simulink model "TrajectoryGenerator3DOF"  (R2023b)
settings: Solver=FixedStepDiscrete  StartTime=0.0  StopTime=1.364*1.4  FixedStep=0.002  RelTol=1e-3
undefined symbols (not defined in the file or in its folder): M_z, Smoothers, Ts
(part 2 of 4)

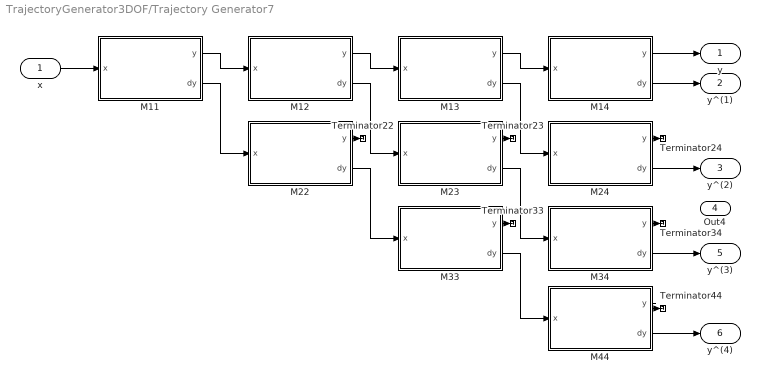
== system TrajectoryGenerator3DOF/Trajectory Generator7 ==
  x : Inport
  M11 : Subsystem  AncestorBlock=Smoothers/M_z  mask{N=643, Ts=0.002, Q0=0}
      mask prompts: N "N_i"; Ts "Sampling period (Ts)"; Q0 "Initial position"
  M12 : Subsystem  AncestorBlock=Smoothers/M_z  mask{N=429, Ts=0.002, Q0=0}
      mask prompts: N "N_i"; Ts "Sampling period (Ts)"; Q0 "Initial position"
  M13 : Subsystem  AncestorBlock=Smoothers/M_z  mask{N=215, Ts=0.002, Q0=0}
      mask prompts: N "N_i"; Ts "Sampling period (Ts)"; Q0 "Initial position"
  M14 : Subsystem  AncestorBlock=Smoothers/M_z  mask{N=215, Ts=0.002, Q0=0}
      mask prompts: N "N_i"; Ts "Sampling period (Ts)"; Q0 "Initial position"
  M22 : Subsystem  AncestorBlock=Smoothers/M_z  mask{N=429, Ts=0.002, Q0=0}
      mask prompts: N "N_i"; Ts "Sampling period (Ts)"; Q0 "Initial position"
  M23 : Subsystem  AncestorBlock=Smoothers/M_z  mask{N=215, Ts=0.002, Q0=0}
      mask prompts: N "N_i"; Ts "Sampling period (Ts)"; Q0 "Initial position"
  M24 : Subsystem  AncestorBlock=Smoothers/M_z  mask{N=215, Ts=0.002, Q0=0}
      mask prompts: N "N_i"; Ts "Sampling period (Ts)"; Q0 "Initial position"
  M33 : Subsystem  AncestorBlock=Smoothers/M_z  mask{N=215, Ts=0.002, Q0=0}
      mask prompts: N "N_i"; Ts "Sampling period (Ts)"; Q0 "Initial position"
  M34 : Subsystem  AncestorBlock=Smoothers/M_z  mask{N=215, Ts=0.002, Q0=0}
      mask prompts: N "N_i"; Ts "Sampling period (Ts)"; Q0 "Initial position"
  M44 : Subsystem  AncestorBlock=Smoothers/M_z  mask{N=215, Ts=0.002, Q0=0}
      mask prompts: N "N_i"; Ts "Sampling period (Ts)"; Q0 "Initial position"
  Terminator{22..24,33..34,44} (6 alike) : Terminator
  y : Outport
  y^(1) : Outport  Port=2
  y^(2) : Outport  Port=3
  Out4 : Outport  Port=4
  y^(3) : Outport  Port=5
  y^(4) : Outport  Port=6
  wires:
  x/1 -> M11/1(x)
  M11/1(y) -> M12/1(x)
  M12/1(y) -> M13/1(x)
  M13/1(y) -> M14/1(x)
  M11/2(dy) -> M22/1(x)
  M12/2(dy) -> M23/1(x)
  M13/2(dy) -> M24/1(x)
  M22/2(dy) -> M33/1(x)
  M23/2(dy) -> M34/1(x)
  M33/2(dy) -> M44/1(x)
  M22/1(y) -> Terminator22/1
  M23/1(y) -> Terminator23/1
  M24/1(y) -> Terminator24/1
  M33/1(y) -> Terminator33/1
  M34/1(y) -> Terminator34/1
  M44/1(y) -> Terminator44/1
  M14/1(y) -> y/1
  M14/2(dy) -> y^(1)/1
  M24/2(dy) -> y^(2)/1
  M34/2(dy) -> y^(3)/1
  M44/2(dy) -> y^(4)/1

== system TrajectoryGenerator3DOF/Trajectory Generator8 ==
  x : Inport
  M11 : Subsystem  AncestorBlock=Smoothers/M_z  mask{N=166, Ts=0.002, Q0=0}
      mask prompts: N "N_i"; Ts "Sampling period (Ts)"; Q0 "Initial position"
  M12 : Subsystem  AncestorBlock=Smoothers/M_z  mask{N=86, Ts=0.002, Q0=0}
      mask prompts: N "N_i"; Ts "Sampling period (Ts)"; Q0 "Initial position"
  M13 : Subsystem  AncestorBlock=Smoothers/M_z  mask{N=43, Ts=0.002, Q0=0}
      mask prompts: N "N_i"; Ts "Sampling period (Ts)"; Q0 "Initial position"
  M14 : Subsystem  AncestorBlock=Smoothers/M_z  mask{N=43, Ts=0.002, Q0=0}
      mask prompts: N "N_i"; Ts "Sampling period (Ts)"; Q0 "Initial position"
  M22 : Subsystem  AncestorBlock=Smoothers/M_z  mask{N=86, Ts=0.002, Q0=0}
      mask prompts: N "N_i"; Ts "Sampling period (Ts)"; Q0 "Initial position"
  M23 : Subsystem  AncestorBlock=Smoothers/M_z  mask{N=43, Ts=0.002, Q0=0}
      mask prompts: N "N_i"; Ts "Sampling period (Ts)"; Q0 "Initial position"
  M24 : Subsystem  AncestorBlock=Smoothers/M_z  mask{N=43, Ts=0.002, Q0=0}
      mask prompts: N "N_i"; Ts "Sampling period (Ts)"; Q0 "Initial position"
  M33 : Subsystem  AncestorBlock=Smoothers/M_z  mask{N=43, Ts=0.002, Q0=0}
      mask prompts: N "N_i"; Ts "Sampling period (Ts)"; Q0 "Initial position"
  M34 : Subsystem  AncestorBlock=Smoothers/M_z  mask{N=43, Ts=0.002, Q0=0}
      mask prompts: N "N_i"; Ts "Sampling period (Ts)"; Q0 "Initial position"
  M44 : Subsystem  AncestorBlock=Smoothers/M_z  mask{N=43, Ts=0.002, Q0=0}
      mask prompts: N "N_i"; Ts "Sampling period (Ts)"; Q0 "Initial position"
  Terminator{22..24,33..34,44} (6 alike) : Terminator
  y : Outport
  y^(1) : Outport  Port=2
  y^(2) : Outport  Port=3
  y^(3) : Outport  Port=4
  y^(4) : Outport  Port=5
  wires:
  x/1 -> M11/1(x)
  M11/1(y) -> M12/1(x)
  M12/1(y) -> M13/1(x)
  M13/1(y) -> M14/1(x)
  M11/2(dy) -> M22/1(x)
  M12/2(dy) -> M23/1(x)
  M13/2(dy) -> M24/1(x)
  M22/2(dy) -> M33/1(x)
  M23/2(dy) -> M34/1(x)
  M33/2(dy) -> M44/1(x)
  M22/1(y) -> Terminator22/1
  M23/1(y) -> Terminator23/1
  M24/1(y) -> Terminator24/1
  M33/1(y) -> Terminator33/1
  M34/1(y) -> Terminator34/1
  M44/1(y) -> Terminator44/1
  M14/1(y) -> y/1
  M14/2(dy) -> y^(1)/1
  M24/2(dy) -> y^(2)/1
  M34/2(dy) -> y^(3)/1
  M44/2(dy) -> y^(4)/1

== system TrajectoryGenerator3DOF/Trajectory Generator9 ==
  x : Inport
  M11 : Subsystem  AncestorBlock=Smoothers/M_z  mask{N=193, Ts=0.002, Q0=0}
      mask prompts: N "N_i"; Ts "Sampling period (Ts)"; Q0 "Initial position"
  M12 : Subsystem  AncestorBlock=Smoothers/M_z  mask{N=166, Ts=0.002, Q0=0}
      mask prompts: N "N_i"; Ts "Sampling period (Ts)"; Q0 "Initial position"
  M13 : Subsystem  AncestorBlock=Smoothers/M_z  mask{N=65, Ts=0.002, Q0=0}
      mask prompts: N "N_i"; Ts "Sampling period (Ts)"; Q0 "Initial position"
  M14 : Subsystem  AncestorBlock=Smoothers/M_z  mask{N=65, Ts=0.002, Q0=0}
      mask prompts: N "N_i"; Ts "Sampling period (Ts)"; Q0 "Initial position"
  M22 : Subsystem  AncestorBlock=Smoothers/M_z  mask{N=166, Ts=0.002, Q0=0}
      mask prompts: N "N_i"; Ts "Sampling period (Ts)"; Q0 "Initial position"
  M23 : Subsystem  AncestorBlock=Smoothers/M_z  mask{N=65, Ts=0.002, Q0=0}
      mask prompts: N "N_i"; Ts "Sampling period (Ts)"; Q0 "Initial position"
  M24 : Subsystem  AncestorBlock=Smoothers/M_z  mask{N=65, Ts=0.002, Q0=0}
      mask prompts: N "N_i"; Ts "Sampling period (Ts)"; Q0 "Initial position"
  M33 : Subsystem  AncestorBlock=Smoothers/M_z  mask{N=65, Ts=0.002, Q0=0}
      mask prompts: N "N_i"; Ts "Sampling period (Ts)"; Q0 "Initial position"
  M34 : Subsystem  AncestorBlock=Smoothers/M_z  mask{N=65, Ts=0.002, Q0=0}
      mask prompts: N "N_i"; Ts "Sampling period (Ts)"; Q0 "Initial position"
  M44 : Subsystem  AncestorBlock=Smoothers/M_z  mask{N=65, Ts=0.002, Q0=0}
      mask prompts: N "N_i"; Ts "Sampling period (Ts)"; Q0 "Initial position"
  Terminator{22..24,33..34,44} (6 alike) : Terminator
  y : Outport
  y^(1) : Outport  Port=2
  y^(2) : Outport  Port=3
  y^(3) : Outport  Port=4
  y^(4) : Outport  Port=5
  wires:
  x/1 -> M11/1(x)
  M11/1(y) -> M12/1(x)
  M12/1(y) -> M13/1(x)
  M13/1(y) -> M14/1(x)
  M11/2(dy) -> M22/1(x)
  M12/2(dy) -> M23/1(x)
  M13/2(dy) -> M24/1(x)
  M22/2(dy) -> M33/1(x)
  M23/2(dy) -> M34/1(x)
  M33/2(dy) -> M44/1(x)
  M22/1(y) -> Terminator22/1
  M23/1(y) -> Terminator23/1
  M24/1(y) -> Terminator24/1
  M33/1(y) -> Terminator33/1
  M34/1(y) -> Terminator34/1
  M44/1(y) -> Terminator44/1
  M14/1(y) -> y/1
  M14/2(dy) -> y^(1)/1
  M24/2(dy) -> y^(2)/1
  M34/2(dy) -> y^(3)/1
  M44/2(dy) -> y^(4)/1

== system TrajectoryGenerator3DOF/Trajectory Generator/M11 ==
  x : Inport
  Discrete FIR Filter1 : DiscreteFir  Coefficients=1/N/Ts*[1 zeros(1,N-1) -1]  InitialStates=Q0  SampleTime=Ts
  Discrete Filter : DiscreteFilter  Numerator=[0 Ts]  Denominator=[1 -1]  InitialStates=Q0  SampleTime=Ts
  y : Outport
  dy : Outport  Port=2
  wires:
  Discrete FIR Filter1/1 -> Discrete Filter/1, dy/1
  x/1 -> Discrete FIR Filter1/1
  Discrete Filter/1 -> y/1

== system TrajectoryGenerator3DOF/Trajectory Generator/M12 ==
  x : Inport
  Discrete FIR Filter1 : DiscreteFir  Coefficients=1/N/Ts*[1 zeros(1,N-1) -1]  InitialStates=Q0  SampleTime=Ts
  Discrete Filter : DiscreteFilter  Numerator=[0 Ts]  Denominator=[1 -1]  InitialStates=Q0  SampleTime=Ts
  y : Outport
  dy : Outport  Port=2
  wires:
  Discrete FIR Filter1/1 -> Discrete Filter/1, dy/1
  x/1 -> Discrete FIR Filter1/1
  Discrete Filter/1 -> y/1

== system TrajectoryGenerator3DOF/Trajectory Generator/M13 ==
  x : Inport
  Discrete FIR Filter1 : DiscreteFir  Coefficients=1/N/Ts*[1 zeros(1,N-1) -1]  InitialStates=Q0  SampleTime=Ts
  Discrete Filter : DiscreteFilter  Numerator=[0 Ts]  Denominator=[1 -1]  InitialStates=Q0  SampleTime=Ts
  y : Outport
  dy : Outport  Port=2
  wires:
  Discrete FIR Filter1/1 -> Discrete Filter/1, dy/1
  x/1 -> Discrete FIR Filter1/1
  Discrete Filter/1 -> y/1

== system TrajectoryGenerator3DOF/Trajectory Generator/M14 ==
  x : Inport
  Discrete FIR Filter1 : DiscreteFir  Coefficients=1/N/Ts*[1 zeros(1,N-1) -1]  InitialStates=Q0  SampleTime=Ts
  Discrete Filter : DiscreteFilter  Numerator=[0 Ts]  Denominator=[1 -1]  InitialStates=Q0  SampleTime=Ts
  y : Outport
  dy : Outport  Port=2
  wires:
  Discrete FIR Filter1/1 -> Discrete Filter/1, dy/1
  x/1 -> Discrete FIR Filter1/1
  Discrete Filter/1 -> y/1

== system TrajectoryGenerator3DOF/Trajectory Generator/M22 ==
  x : Inport
  Discrete FIR Filter1 : DiscreteFir  Coefficients=1/N/Ts*[1 zeros(1,N-1) -1]  InitialStates=Q0  SampleTime=Ts
  Discrete Filter : DiscreteFilter  Numerator=[0 Ts]  Denominator=[1 -1]  InitialStates=Q0  SampleTime=Ts
  y : Outport
  dy : Outport  Port=2
  wires:
  Discrete FIR Filter1/1 -> Discrete Filter/1, dy/1
  x/1 -> Discrete FIR Filter1/1
  Discrete Filter/1 -> y/1

== system TrajectoryGenerator3DOF/Trajectory Generator/M23 ==
  x : Inport
  Discrete FIR Filter1 : DiscreteFir  Coefficients=1/N/Ts*[1 zeros(1,N-1) -1]  InitialStates=Q0  SampleTime=Ts
  Discrete Filter : DiscreteFilter  Numerator=[0 Ts]  Denominator=[1 -1]  InitialStates=Q0  SampleTime=Ts
  y : Outport
  dy : Outport  Port=2
  wires:
  Discrete FIR Filter1/1 -> Discrete Filter/1, dy/1
  x/1 -> Discrete FIR Filter1/1
  Discrete Filter/1 -> y/1

== system TrajectoryGenerator3DOF/Trajectory Generator/M24 ==
  x : Inport
  Discrete FIR Filter1 : DiscreteFir  Coefficients=1/N/Ts*[1 zeros(1,N-1) -1]  InitialStates=Q0  SampleTime=Ts
  Discrete Filter : DiscreteFilter  Numerator=[0 Ts]  Denominator=[1 -1]  InitialStates=Q0  SampleTime=Ts
  y : Outport
  dy : Outport  Port=2
  wires:
  Discrete FIR Filter1/1 -> Discrete Filter/1, dy/1
  x/1 -> Discrete FIR Filter1/1
  Discrete Filter/1 -> y/1

== system TrajectoryGenerator3DOF/Trajectory Generator/M33 ==
  x : Inport
  Discrete FIR Filter1 : DiscreteFir  Coefficients=1/N/Ts*[1 zeros(1,N-1) -1]  InitialStates=Q0  SampleTime=Ts
  Discrete Filter : DiscreteFilter  Numerator=[0 Ts]  Denominator=[1 -1]  InitialStates=Q0  SampleTime=Ts
  y : Outport
  dy : Outport  Port=2
  wires:
  Discrete FIR Filter1/1 -> Discrete Filter/1, dy/1
  x/1 -> Discrete FIR Filter1/1
  Discrete Filter/1 -> y/1

== system TrajectoryGenerator3DOF/Trajectory Generator/M34 ==
  x : Inport
  Discrete FIR Filter1 : DiscreteFir  Coefficients=1/N/Ts*[1 zeros(1,N-1) -1]  InitialStates=Q0  SampleTime=Ts
  Discrete Filter : DiscreteFilter  Numerator=[0 Ts]  Denominator=[1 -1]  InitialStates=Q0  SampleTime=Ts
  y : Outport
  dy : Outport  Port=2
  wires:
  Discrete FIR Filter1/1 -> Discrete Filter/1, dy/1
  x/1 -> Discrete FIR Filter1/1
  Discrete Filter/1 -> y/1

== system TrajectoryGenerator3DOF/Trajectory Generator/M44 ==
  x : Inport
  Discrete FIR Filter1 : DiscreteFir  Coefficients=1/N/Ts*[1 zeros(1,N-1) -1]  InitialStates=Q0  SampleTime=Ts
  Discrete Filter : DiscreteFilter  Numerator=[0 Ts]  Denominator=[1 -1]  InitialStates=Q0  SampleTime=Ts
  y : Outport
  dy : Outport  Port=2
  wires:
  Discrete FIR Filter1/1 -> Discrete Filter/1, dy/1
  x/1 -> Discrete FIR Filter1/1
  Discrete Filter/1 -> y/1

== system TrajectoryGenerator3DOF/Trajectory Generator1/M11 ==
  x : Inport
  Discrete FIR Filter1 : DiscreteFir  Coefficients=1/N/Ts*[1 zeros(1,N-1) -1]  InitialStates=Q0  SampleTime=Ts
  Discrete Filter : DiscreteFilter  Numerator=[0 Ts]  Denominator=[1 -1]  InitialStates=Q0  SampleTime=Ts
  y : Outport
  dy : Outport  Port=2
  wires:
  Discrete Filter/1 -> y/1
  x/1 -> Discrete FIR Filter1/1
  Discrete FIR Filter1/1 -> dy/1, Discrete Filter/1

== system TrajectoryGenerator3DOF/Trajectory Generator1/M12 ==
  x : Inport
  Discrete FIR Filter1 : DiscreteFir  Coefficients=1/N/Ts*[1 zeros(1,N-1) -1]  InitialStates=Q0  SampleTime=Ts
  Discrete Filter : DiscreteFilter  Numerator=[0 Ts]  Denominator=[1 -1]  InitialStates=Q0  SampleTime=Ts
  y : Outport
  dy : Outport  Port=2
  wires:
  Discrete Filter/1 -> y/1
  x/1 -> Discrete FIR Filter1/1
  Discrete FIR Filter1/1 -> dy/1, Discrete Filter/1

== system TrajectoryGenerator3DOF/Trajectory Generator1/M13 ==
  x : Inport
  Discrete FIR Filter1 : DiscreteFir  Coefficients=1/N/Ts*[1 zeros(1,N-1) -1]  InitialStates=Q0  SampleTime=Ts
  Discrete Filter : DiscreteFilter  Numerator=[0 Ts]  Denominator=[1 -1]  InitialStates=Q0  SampleTime=Ts
  y : Outport
  dy : Outport  Port=2
  wires:
  Discrete Filter/1 -> y/1
  x/1 -> Discrete FIR Filter1/1
  Discrete FIR Filter1/1 -> dy/1, Discrete Filter/1

== system TrajectoryGenerator3DOF/Trajectory Generator1/M14 ==
  x : Inport
  Discrete FIR Filter1 : DiscreteFir  Coefficients=1/N/Ts*[1 zeros(1,N-1) -1]  InitialStates=Q0  SampleTime=Ts
  Discrete Filter : DiscreteFilter  Numerator=[0 Ts]  Denominator=[1 -1]  InitialStates=Q0  SampleTime=Ts
  y : Outport
  dy : Outport  Port=2
  wires:
  Discrete Filter/1 -> y/1
  x/1 -> Discrete FIR Filter1/1
  Discrete FIR Filter1/1 -> dy/1, Discrete Filter/1

== system TrajectoryGenerator3DOF/Trajectory Generator1/M22 ==
  x : Inport
  Discrete FIR Filter1 : DiscreteFir  Coefficients=1/N/Ts*[1 zeros(1,N-1) -1]  InitialStates=Q0  SampleTime=Ts
  Discrete Filter : DiscreteFilter  Numerator=[0 Ts]  Denominator=[1 -1]  InitialStates=Q0  SampleTime=Ts
  y : Outport
  dy : Outport  Port=2
  wires:
  Discrete Filter/1 -> y/1
  x/1 -> Discrete FIR Filter1/1
  Discrete FIR Filter1/1 -> dy/1, Discrete Filter/1

== system TrajectoryGenerator3DOF/Trajectory Generator1/M23 ==
  x : Inport
  Discrete FIR Filter1 : DiscreteFir  Coefficients=1/N/Ts*[1 zeros(1,N-1) -1]  InitialStates=Q0  SampleTime=Ts
  Discrete Filter : DiscreteFilter  Numerator=[0 Ts]  Denominator=[1 -1]  InitialStates=Q0  SampleTime=Ts
  y : Outport
  dy : Outport  Port=2
  wires:
  Discrete Filter/1 -> y/1
  x/1 -> Discrete FIR Filter1/1
  Discrete FIR Filter1/1 -> dy/1, Discrete Filter/1

== system TrajectoryGenerator3DOF/Trajectory Generator1/M24 ==
  x : Inport
  Discrete FIR Filter1 : DiscreteFir  Coefficients=1/N/Ts*[1 zeros(1,N-1) -1]  InitialStates=Q0  SampleTime=Ts
  Discrete Filter : DiscreteFilter  Numerator=[0 Ts]  Denominator=[1 -1]  InitialStates=Q0  SampleTime=Ts
  y : Outport
  dy : Outport  Port=2
  wires:
  Discrete Filter/1 -> y/1
  x/1 -> Discrete FIR Filter1/1
  Discrete FIR Filter1/1 -> dy/1, Discrete Filter/1

== system TrajectoryGenerator3DOF/Trajectory Generator1/M33 ==
  x : Inport
  Discrete FIR Filter1 : DiscreteFir  Coefficients=1/N/Ts*[1 zeros(1,N-1) -1]  InitialStates=Q0  SampleTime=Ts
  Discrete Filter : DiscreteFilter  Numerator=[0 Ts]  Denominator=[1 -1]  InitialStates=Q0  SampleTime=Ts
  y : Outport
  dy : Outport  Port=2
  wires:
  Discrete Filter/1 -> y/1
  x/1 -> Discrete FIR Filter1/1
  Discrete FIR Filter1/1 -> dy/1, Discrete Filter/1

== system TrajectoryGenerator3DOF/Trajectory Generator1/M34 ==
  x : Inport
  Discrete FIR Filter1 : DiscreteFir  Coefficients=1/N/Ts*[1 zeros(1,N-1) -1]  InitialStates=Q0  SampleTime=Ts
  Discrete Filter : DiscreteFilter  Numerator=[0 Ts]  Denominator=[1 -1]  InitialStates=Q0  SampleTime=Ts
  y : Outport
  dy : Outport  Port=2
  wires:
  Discrete Filter/1 -> y/1
  x/1 -> Discrete FIR Filter1/1
  Discrete FIR Filter1/1 -> dy/1, Discrete Filter/1

== system TrajectoryGenerator3DOF/Trajectory Generator1/M44 ==
  x : Inport
  Discrete FIR Filter1 : DiscreteFir  Coefficients=1/N/Ts*[1 zeros(1,N-1) -1]  InitialStates=Q0  SampleTime=Ts
  Discrete Filter : DiscreteFilter  Numerator=[0 Ts]  Denominator=[1 -1]  InitialStates=Q0  SampleTime=Ts
  y : Outport
  dy : Outport  Port=2
  wires:
  Discrete Filter/1 -> y/1
  x/1 -> Discrete FIR Filter1/1
  Discrete FIR Filter1/1 -> dy/1, Discrete Filter/1

== system TrajectoryGenerator3DOF/Trajectory Generator10/M11 ==
  x : Inport
  Discrete FIR Filter1 : DiscreteFir  Coefficients=1/N/Ts*[1 zeros(1,N-1) -1]  InitialStates=Q0  SampleTime=Ts
  Discrete Filter : DiscreteFilter  Numerator=[0 Ts]  Denominator=[1 -1]  InitialStates=Q0  SampleTime=Ts
  y : Outport
  dy : Outport  Port=2
  wires:
  Discrete FIR Filter1/1 -> Discrete Filter/1, dy/1
  x/1 -> Discrete FIR Filter1/1
  Discrete Filter/1 -> y/1

== system TrajectoryGenerator3DOF/Trajectory Generator10/M12 ==
  x : Inport
  Discrete FIR Filter1 : DiscreteFir  Coefficients=1/N/Ts*[1 zeros(1,N-1) -1]  InitialStates=Q0  SampleTime=Ts
  Discrete Filter : DiscreteFilter  Numerator=[0 Ts]  Denominator=[1 -1]  InitialStates=Q0  SampleTime=Ts
  y : Outport
  dy : Outport  Port=2
  wires:
  Discrete FIR Filter1/1 -> Discrete Filter/1, dy/1
  x/1 -> Discrete FIR Filter1/1
  Discrete Filter/1 -> y/1

== system TrajectoryGenerator3DOF/Trajectory Generator10/M13 ==
  x : Inport
  Discrete FIR Filter1 : DiscreteFir  Coefficients=1/N/Ts*[1 zeros(1,N-1) -1]  InitialStates=Q0  SampleTime=Ts
  Discrete Filter : DiscreteFilter  Numerator=[0 Ts]  Denominator=[1 -1]  InitialStates=Q0  SampleTime=Ts
  y : Outport
  dy : Outport  Port=2
  wires:
  Discrete FIR Filter1/1 -> Discrete Filter/1, dy/1
  x/1 -> Discrete FIR Filter1/1
  Discrete Filter/1 -> y/1

== system TrajectoryGenerator3DOF/Trajectory Generator10/M14 ==
  x : Inport
  Discrete FIR Filter1 : DiscreteFir  Coefficients=1/N/Ts*[1 zeros(1,N-1) -1]  InitialStates=Q0  SampleTime=Ts
  Discrete Filter : DiscreteFilter  Numerator=[0 Ts]  Denominator=[1 -1]  InitialStates=Q0  SampleTime=Ts
  y : Outport
  dy : Outport  Port=2
  wires:
  Discrete FIR Filter1/1 -> Discrete Filter/1, dy/1
  x/1 -> Discrete FIR Filter1/1
  Discrete Filter/1 -> y/1

== system TrajectoryGenerator3DOF/Trajectory Generator10/M22 ==
  x : Inport
  Discrete FIR Filter1 : DiscreteFir  Coefficients=1/N/Ts*[1 zeros(1,N-1) -1]  InitialStates=Q0  SampleTime=Ts
  Discrete Filter : DiscreteFilter  Numerator=[0 Ts]  Denominator=[1 -1]  InitialStates=Q0  SampleTime=Ts
  y : Outport
  dy : Outport  Port=2
  wires:
  Discrete FIR Filter1/1 -> Discrete Filter/1, dy/1
  x/1 -> Discrete FIR Filter1/1
  Discrete Filter/1 -> y/1

== system TrajectoryGenerator3DOF/Trajectory Generator10/M23 ==
  x : Inport
  Discrete FIR Filter1 : DiscreteFir  Coefficients=1/N/Ts*[1 zeros(1,N-1) -1]  InitialStates=Q0  SampleTime=Ts
  Discrete Filter : DiscreteFilter  Numerator=[0 Ts]  Denominator=[1 -1]  InitialStates=Q0  SampleTime=Ts
  y : Outport
  dy : Outport  Port=2
  wires:
  Discrete FIR Filter1/1 -> Discrete Filter/1, dy/1
  x/1 -> Discrete FIR Filter1/1
  Discrete Filter/1 -> y/1

== system TrajectoryGenerator3DOF/Trajectory Generator10/M24 ==
  x : Inport
  Discrete FIR Filter1 : DiscreteFir  Coefficients=1/N/Ts*[1 zeros(1,N-1) -1]  InitialStates=Q0  SampleTime=Ts
  Discrete Filter : DiscreteFilter  Numerator=[0 Ts]  Denominator=[1 -1]  InitialStates=Q0  SampleTime=Ts
  y : Outport
  dy : Outport  Port=2
  wires:
  Discrete FIR Filter1/1 -> Discrete Filter/1, dy/1
  x/1 -> Discrete FIR Filter1/1
  Discrete Filter/1 -> y/1

== system TrajectoryGenerator3DOF/Trajectory Generator10/M33 ==
  x : Inport
  Discrete FIR Filter1 : DiscreteFir  Coefficients=1/N/Ts*[1 zeros(1,N-1) -1]  InitialStates=Q0  SampleTime=Ts
  Discrete Filter : DiscreteFilter  Numerator=[0 Ts]  Denominator=[1 -1]  InitialStates=Q0  SampleTime=Ts
  y : Outport
  dy : Outport  Port=2
  wires:
  Discrete FIR Filter1/1 -> Discrete Filter/1, dy/1
  x/1 -> Discrete FIR Filter1/1
  Discrete Filter/1 -> y/1

== system TrajectoryGenerator3DOF/Trajectory Generator10/M34 ==
  x : Inport
  Discrete FIR Filter1 : DiscreteFir  Coefficients=1/N/Ts*[1 zeros(1,N-1) -1]  InitialStates=Q0  SampleTime=Ts
  Discrete Filter : DiscreteFilter  Numerator=[0 Ts]  Denominator=[1 -1]  InitialStates=Q0  SampleTime=Ts
  y : Outport
  dy : Outport  Port=2
  wires:
  Discrete FIR Filter1/1 -> Discrete Filter/1, dy/1
  x/1 -> Discrete FIR Filter1/1
  Discrete Filter/1 -> y/1

== system TrajectoryGenerator3DOF/Trajectory Generator10/M44 ==
  x : Inport
  Discrete FIR Filter1 : DiscreteFir  Coefficients=1/N/Ts*[1 zeros(1,N-1) -1]  InitialStates=Q0  SampleTime=Ts
  Discrete Filter : DiscreteFilter  Numerator=[0 Ts]  Denominator=[1 -1]  InitialStates=Q0  SampleTime=Ts
  y : Outport
  dy : Outport  Port=2
  wires:
  Discrete FIR Filter1/1 -> Discrete Filter/1, dy/1
  x/1 -> Discrete FIR Filter1/1
  Discrete Filter/1 -> y/1

== system TrajectoryGenerator3DOF/Trajectory Generator11/M11 ==
  x : Inport
  Discrete FIR Filter1 : DiscreteFir  Coefficients=1/N/Ts*[1 zeros(1,N-1) -1]  InitialStates=Q0  SampleTime=Ts
  Discrete Filter : DiscreteFilter  Numerator=[0 Ts]  Denominator=[1 -1]  InitialStates=Q0  SampleTime=Ts
  y : Outport
  dy : Outport  Port=2
  wires:
  Discrete FIR Filter1/1 -> Discrete Filter/1, dy/1
  x/1 -> Discrete FIR Filter1/1
  Discrete Filter/1 -> y/1

== system TrajectoryGenerator3DOF/Trajectory Generator11/M12 ==
  x : Inport
  Discrete FIR Filter1 : DiscreteFir  Coefficients=1/N/Ts*[1 zeros(1,N-1) -1]  InitialStates=Q0  SampleTime=Ts
  Discrete Filter : DiscreteFilter  Numerator=[0 Ts]  Denominator=[1 -1]  InitialStates=Q0  SampleTime=Ts
  y : Outport
  dy : Outport  Port=2
  wires:
  Discrete FIR Filter1/1 -> Discrete Filter/1, dy/1
  x/1 -> Discrete FIR Filter1/1
  Discrete Filter/1 -> y/1

== system TrajectoryGenerator3DOF/Trajectory Generator11/M13 ==
  x : Inport
  Discrete FIR Filter1 : DiscreteFir  Coefficients=1/N/Ts*[1 zeros(1,N-1) -1]  InitialStates=Q0  SampleTime=Ts
  Discrete Filter : DiscreteFilter  Numerator=[0 Ts]  Denominator=[1 -1]  InitialStates=Q0  SampleTime=Ts
  y : Outport
  dy : Outport  Port=2
  wires:
  Discrete FIR Filter1/1 -> Discrete Filter/1, dy/1
  x/1 -> Discrete FIR Filter1/1
  Discrete Filter/1 -> y/1

== system TrajectoryGenerator3DOF/Trajectory Generator11/M14 ==
  x : Inport
  Discrete FIR Filter1 : DiscreteFir  Coefficients=1/N/Ts*[1 zeros(1,N-1) -1]  InitialStates=Q0  SampleTime=Ts
  Discrete Filter : DiscreteFilter  Numerator=[0 Ts]  Denominator=[1 -1]  InitialStates=Q0  SampleTime=Ts
  y : Outport
  dy : Outport  Port=2
  wires:
  Discrete FIR Filter1/1 -> Discrete Filter/1, dy/1
  x/1 -> Discrete FIR Filter1/1
  Discrete Filter/1 -> y/1

== system TrajectoryGenerator3DOF/Trajectory Generator11/M22 ==
  x : Inport
  Discrete FIR Filter1 : DiscreteFir  Coefficients=1/N/Ts*[1 zeros(1,N-1) -1]  InitialStates=Q0  SampleTime=Ts
  Discrete Filter : DiscreteFilter  Numerator=[0 Ts]  Denominator=[1 -1]  InitialStates=Q0  SampleTime=Ts
  y : Outport
  dy : Outport  Port=2
  wires:
  Discrete FIR Filter1/1 -> Discrete Filter/1, dy/1
  x/1 -> Discrete FIR Filter1/1
  Discrete Filter/1 -> y/1

== system TrajectoryGenerator3DOF/Trajectory Generator11/M23 ==
  x : Inport
  Discrete FIR Filter1 : DiscreteFir  Coefficients=1/N/Ts*[1 zeros(1,N-1) -1]  InitialStates=Q0  SampleTime=Ts
  Discrete Filter : DiscreteFilter  Numerator=[0 Ts]  Denominator=[1 -1]  InitialStates=Q0  SampleTime=Ts
  y : Outport
  dy : Outport  Port=2
  wires:
  Discrete FIR Filter1/1 -> Discrete Filter/1, dy/1
  x/1 -> Discrete FIR Filter1/1
  Discrete Filter/1 -> y/1

== system TrajectoryGenerator3DOF/Trajectory Generator11/M24 ==
  x : Inport
  Discrete FIR Filter1 : DiscreteFir  Coefficients=1/N/Ts*[1 zeros(1,N-1) -1]  InitialStates=Q0  SampleTime=Ts
  Discrete Filter : DiscreteFilter  Numerator=[0 Ts]  Denominator=[1 -1]  InitialStates=Q0  SampleTime=Ts
  y : Outport
  dy : Outport  Port=2
  wires:
  Discrete FIR Filter1/1 -> Discrete Filter/1, dy/1
  x/1 -> Discrete FIR Filter1/1
  Discrete Filter/1 -> y/1

== system TrajectoryGenerator3DOF/Trajectory Generator11/M33 ==
  x : Inport
  Discrete FIR Filter1 : DiscreteFir  Coefficients=1/N/Ts*[1 zeros(1,N-1) -1]  InitialStates=Q0  SampleTime=Ts
  Discrete Filter : DiscreteFilter  Numerator=[0 Ts]  Denominator=[1 -1]  InitialStates=Q0  SampleTime=Ts
  y : Outport
  dy : Outport  Port=2
  wires:
  Discrete FIR Filter1/1 -> Discrete Filter/1, dy/1
  x/1 -> Discrete FIR Filter1/1
  Discrete Filter/1 -> y/1

== system TrajectoryGenerator3DOF/Trajectory Generator11/M34 ==
  x : Inport
  Discrete FIR Filter1 : DiscreteFir  Coefficients=1/N/Ts*[1 zeros(1,N-1) -1]  InitialStates=Q0  SampleTime=Ts
  Discrete Filter : DiscreteFilter  Numerator=[0 Ts]  Denominator=[1 -1]  InitialStates=Q0  SampleTime=Ts
  y : Outport
  dy : Outport  Port=2
  wires:
  Discrete FIR Filter1/1 -> Discrete Filter/1, dy/1
  x/1 -> Discrete FIR Filter1/1
  Discrete Filter/1 -> y/1

== system TrajectoryGenerator3DOF/Trajectory Generator11/M44 ==
  x : Inport
  Discrete FIR Filter1 : DiscreteFir  Coefficients=1/N/Ts*[1 zeros(1,N-1) -1]  InitialStates=Q0  SampleTime=Ts
  Discrete Filter : DiscreteFilter  Numerator=[0 Ts]  Denominator=[1 -1]  InitialStates=Q0  SampleTime=Ts
  y : Outport
  dy : Outport  Port=2
  wires:
  Discrete FIR Filter1/1 -> Discrete Filter/1, dy/1
  x/1 -> Discrete FIR Filter1/1
  Discrete Filter/1 -> y/1

== system TrajectoryGenerator3DOF/Trajectory Generator12/M11 ==
  x : Inport
  Discrete FIR Filter1 : DiscreteFir  Coefficients=1/N/Ts*[1 zeros(1,N-1) -1]  InitialStates=Q0  SampleTime=Ts
  Discrete Filter : DiscreteFilter  Numerator=[0 Ts]  Denominator=[1 -1]  InitialStates=Q0  SampleTime=Ts
  y : Outport
  dy : Outport  Port=2
  wires:
  Discrete FIR Filter1/1 -> Discrete Filter/1, dy/1
  x/1 -> Discrete FIR Filter1/1
  Discrete Filter/1 -> y/1

== system TrajectoryGenerator3DOF/Trajectory Generator12/M12 ==
  x : Inport
  Discrete FIR Filter1 : DiscreteFir  Coefficients=1/N/Ts*[1 zeros(1,N-1) -1]  InitialStates=Q0  SampleTime=Ts
  Discrete Filter : DiscreteFilter  Numerator=[0 Ts]  Denominator=[1 -1]  InitialStates=Q0  SampleTime=Ts
  y : Outport
  dy : Outport  Port=2
  wires:
  Discrete FIR Filter1/1 -> Discrete Filter/1, dy/1
  x/1 -> Discrete FIR Filter1/1
  Discrete Filter/1 -> y/1

== system TrajectoryGenerator3DOF/Trajectory Generator12/M13 ==
  x : Inport
  Discrete FIR Filter1 : DiscreteFir  Coefficients=1/N/Ts*[1 zeros(1,N-1) -1]  InitialStates=Q0  SampleTime=Ts
  Discrete Filter : DiscreteFilter  Numerator=[0 Ts]  Denominator=[1 -1]  InitialStates=Q0  SampleTime=Ts
  y : Outport
  dy : Outport  Port=2
  wires:
  Discrete FIR Filter1/1 -> Discrete Filter/1, dy/1
  x/1 -> Discrete FIR Filter1/1
  Discrete Filter/1 -> y/1

== system TrajectoryGenerator3DOF/Trajectory Generator12/M14 ==
  x : Inport
  Discrete FIR Filter1 : DiscreteFir  Coefficients=1/N/Ts*[1 zeros(1,N-1) -1]  InitialStates=Q0  SampleTime=Ts
  Discrete Filter : DiscreteFilter  Numerator=[0 Ts]  Denominator=[1 -1]  InitialStates=Q0  SampleTime=Ts
  y : Outport
  dy : Outport  Port=2
  wires:
  Discrete FIR Filter1/1 -> Discrete Filter/1, dy/1
  x/1 -> Discrete FIR Filter1/1
  Discrete Filter/1 -> y/1

== system TrajectoryGenerator3DOF/Trajectory Generator12/M22 ==
  x : Inport
  Discrete FIR Filter1 : DiscreteFir  Coefficients=1/N/Ts*[1 zeros(1,N-1) -1]  InitialStates=Q0  SampleTime=Ts
  Discrete Filter : DiscreteFilter  Numerator=[0 Ts]  Denominator=[1 -1]  InitialStates=Q0  SampleTime=Ts
  y : Outport
  dy : Outport  Port=2
  wires:
  Discrete FIR Filter1/1 -> Discrete Filter/1, dy/1
  x/1 -> Discrete FIR Filter1/1
  Discrete Filter/1 -> y/1

== system TrajectoryGenerator3DOF/Trajectory Generator12/M23 ==
  x : Inport
  Discrete FIR Filter1 : DiscreteFir  Coefficients=1/N/Ts*[1 zeros(1,N-1) -1]  InitialStates=Q0  SampleTime=Ts
  Discrete Filter : DiscreteFilter  Numerator=[0 Ts]  Denominator=[1 -1]  InitialStates=Q0  SampleTime=Ts
  y : Outport
  dy : Outport  Port=2
  wires:
  Discrete FIR Filter1/1 -> Discrete Filter/1, dy/1
  x/1 -> Discrete FIR Filter1/1
  Discrete Filter/1 -> y/1

== system TrajectoryGenerator3DOF/Trajectory Generator12/M24 ==
  x : Inport
  Discrete FIR Filter1 : DiscreteFir  Coefficients=1/N/Ts*[1 zeros(1,N-1) -1]  InitialStates=Q0  SampleTime=Ts
  Discrete Filter : DiscreteFilter  Numerator=[0 Ts]  Denominator=[1 -1]  InitialStates=Q0  SampleTime=Ts
  y : Outport
  dy : Outport  Port=2
  wires:
  Discrete FIR Filter1/1 -> Discrete Filter/1, dy/1
  x/1 -> Discrete FIR Filter1/1
  Discrete Filter/1 -> y/1

== system TrajectoryGenerator3DOF/Trajectory Generator12/M33 ==
  x : Inport
  Discrete FIR Filter1 : DiscreteFir  Coefficients=1/N/Ts*[1 zeros(1,N-1) -1]  InitialStates=Q0  SampleTime=Ts
  Discrete Filter : DiscreteFilter  Numerator=[0 Ts]  Denominator=[1 -1]  InitialStates=Q0  SampleTime=Ts
  y : Outport
  dy : Outport  Port=2
  wires:
  Discrete FIR Filter1/1 -> Discrete Filter/1, dy/1
  x/1 -> Discrete FIR Filter1/1
  Discrete Filter/1 -> y/1

== system TrajectoryGenerator3DOF/Trajectory Generator12/M34 ==
  x : Inport
  Discrete FIR Filter1 : DiscreteFir  Coefficients=1/N/Ts*[1 zeros(1,N-1) -1]  InitialStates=Q0  SampleTime=Ts
  Discrete Filter : DiscreteFilter  Numerator=[0 Ts]  Denominator=[1 -1]  InitialStates=Q0  SampleTime=Ts
  y : Outport
  dy : Outport  Port=2
  wires:
  Discrete FIR Filter1/1 -> Discrete Filter/1, dy/1
  x/1 -> Discrete FIR Filter1/1
  Discrete Filter/1 -> y/1

== system TrajectoryGenerator3DOF/Trajectory Generator12/M44 ==
  x : Inport
  Discrete FIR Filter1 : DiscreteFir  Coefficients=1/N/Ts*[1 zeros(1,N-1) -1]  InitialStates=Q0  SampleTime=Ts
  Discrete Filter : DiscreteFilter  Numerator=[0 Ts]  Denominator=[1 -1]  InitialStates=Q0  SampleTime=Ts
  y : Outport
  dy : Outport  Port=2
  wires:
  Discrete FIR Filter1/1 -> Discrete Filter/1, dy/1
  x/1 -> Discrete FIR Filter1/1
  Discrete Filter/1 -> y/1

== system TrajectoryGenerator3DOF/Trajectory Generator13/M11 ==
  x : Inport
  Discrete FIR Filter1 : DiscreteFir  Coefficients=1/N/Ts*[1 zeros(1,N-1) -1]  InitialStates=Q0  SampleTime=Ts
  Discrete Filter : DiscreteFilter  Numerator=[0 Ts]  Denominator=[1 -1]  InitialStates=Q0  SampleTime=Ts
  y : Outport
  dy : Outport  Port=2
  wires:
  Discrete FIR Filter1/1 -> Discrete Filter/1, dy/1
  x/1 -> Discrete FIR Filter1/1
  Discrete Filter/1 -> y/1

== system TrajectoryGenerator3DOF/Trajectory Generator13/M12 ==
  x : Inport
  Discrete FIR Filter1 : DiscreteFir  Coefficients=1/N/Ts*[1 zeros(1,N-1) -1]  InitialStates=Q0  SampleTime=Ts
  Discrete Filter : DiscreteFilter  Numerator=[0 Ts]  Denominator=[1 -1]  InitialStates=Q0  SampleTime=Ts
  y : Outport
  dy : Outport  Port=2
  wires:
  Discrete FIR Filter1/1 -> Discrete Filter/1, dy/1
  x/1 -> Discrete FIR Filter1/1
  Discrete Filter/1 -> y/1

== system TrajectoryGenerator3DOF/Trajectory Generator13/M13 ==
  x : Inport
  Discrete FIR Filter1 : DiscreteFir  Coefficients=1/N/Ts*[1 zeros(1,N-1) -1]  InitialStates=Q0  SampleTime=Ts
  Discrete Filter : DiscreteFilter  Numerator=[0 Ts]  Denominator=[1 -1]  InitialStates=Q0  SampleTime=Ts
  y : Outport
  dy : Outport  Port=2
  wires:
  Discrete FIR Filter1/1 -> Discrete Filter/1, dy/1
  x/1 -> Discrete FIR Filter1/1
  Discrete Filter/1 -> y/1

== system TrajectoryGenerator3DOF/Trajectory Generator13/M14 ==
  x : Inport
  Discrete FIR Filter1 : DiscreteFir  Coefficients=1/N/Ts*[1 zeros(1,N-1) -1]  InitialStates=Q0  SampleTime=Ts
  Discrete Filter : DiscreteFilter  Numerator=[0 Ts]  Denominator=[1 -1]  InitialStates=Q0  SampleTime=Ts
  y : Outport
  dy : Outport  Port=2
  wires:
  Discrete FIR Filter1/1 -> Discrete Filter/1, dy/1
  x/1 -> Discrete FIR Filter1/1
  Discrete Filter/1 -> y/1

== system TrajectoryGenerator3DOF/Trajectory Generator13/M22 ==
  x : Inport
  Discrete FIR Filter1 : DiscreteFir  Coefficients=1/N/Ts*[1 zeros(1,N-1) -1]  InitialStates=Q0  SampleTime=Ts
  Discrete Filter : DiscreteFilter  Numerator=[0 Ts]  Denominator=[1 -1]  InitialStates=Q0  SampleTime=Ts
  y : Outport
  dy : Outport  Port=2
  wires:
  Discrete FIR Filter1/1 -> Discrete Filter/1, dy/1
  x/1 -> Discrete FIR Filter1/1
  Discrete Filter/1 -> y/1

== system TrajectoryGenerator3DOF/Trajectory Generator13/M23 ==
  x : Inport
  Discrete FIR Filter1 : DiscreteFir  Coefficients=1/N/Ts*[1 zeros(1,N-1) -1]  InitialStates=Q0  SampleTime=Ts
  Discrete Filter : DiscreteFilter  Numerator=[0 Ts]  Denominator=[1 -1]  InitialStates=Q0  SampleTime=Ts
  y : Outport
  dy : Outport  Port=2
  wires:
  Discrete FIR Filter1/1 -> Discrete Filter/1, dy/1
  x/1 -> Discrete FIR Filter1/1
  Discrete Filter/1 -> y/1

== system TrajectoryGenerator3DOF/Trajectory Generator13/M24 ==
  x : Inport
  Discrete FIR Filter1 : DiscreteFir  Coefficients=1/N/Ts*[1 zeros(1,N-1) -1]  InitialStates=Q0  SampleTime=Ts
  Discrete Filter : DiscreteFilter  Numerator=[0 Ts]  Denominator=[1 -1]  InitialStates=Q0  SampleTime=Ts
  y : Outport
  dy : Outport  Port=2
  wires:
  Discrete FIR Filter1/1 -> Discrete Filter/1, dy/1
  x/1 -> Discrete FIR Filter1/1
  Discrete Filter/1 -> y/1

== system TrajectoryGenerator3DOF/Trajectory Generator13/M33 ==
  x : Inport
  Discrete FIR Filter1 : DiscreteFir  Coefficients=1/N/Ts*[1 zeros(1,N-1) -1]  InitialStates=Q0  SampleTime=Ts
  Discrete Filter : DiscreteFilter  Numerator=[0 Ts]  Denominator=[1 -1]  InitialStates=Q0  SampleTime=Ts
  y : Outport
  dy : Outport  Port=2
  wires:
  Discrete FIR Filter1/1 -> Discrete Filter/1, dy/1
  x/1 -> Discrete FIR Filter1/1
  Discrete Filter/1 -> y/1

== system TrajectoryGenerator3DOF/Trajectory Generator13/M34 ==
  x : Inport
  Discrete FIR Filter1 : DiscreteFir  Coefficients=1/N/Ts*[1 zeros(1,N-1) -1]  InitialStates=Q0  SampleTime=Ts
  Discrete Filter : DiscreteFilter  Numerator=[0 Ts]  Denominator=[1 -1]  InitialStates=Q0  SampleTime=Ts
  y : Outport
  dy : Outport  Port=2
  wires:
  Discrete FIR Filter1/1 -> Discrete Filter/1, dy/1
  x/1 -> Discrete FIR Filter1/1
  Discrete Filter/1 -> y/1

== system TrajectoryGenerator3DOF/Trajectory Generator13/M44 ==
  x : Inport
  Discrete FIR Filter1 : DiscreteFir  Coefficients=1/N/Ts*[1 zeros(1,N-1) -1]  InitialStates=Q0  SampleTime=Ts
  Discrete Filter : DiscreteFilter  Numerator=[0 Ts]  Denominator=[1 -1]  InitialStates=Q0  SampleTime=Ts
  y : Outport
  dy : Outport  Port=2
  wires:
  Discrete FIR Filter1/1 -> Discrete Filter/1, dy/1
  x/1 -> Discrete FIR Filter1/1
  Discrete Filter/1 -> y/1

== system TrajectoryGenerator3DOF/Trajectory Generator14/M11 ==
  x : Inport
  Discrete FIR Filter1 : DiscreteFir  Coefficients=1/N/Ts*[1 zeros(1,N-1) -1]  InitialStates=Q0  SampleTime=Ts
  Discrete Filter : DiscreteFilter  Numerator=[0 Ts]  Denominator=[1 -1]  InitialStates=Q0  SampleTime=Ts
  y : Outport
  dy : Outport  Port=2
  wires:
  Discrete FIR Filter1/1 -> Discrete Filter/1, dy/1
  x/1 -> Discrete FIR Filter1/1
  Discrete Filter/1 -> y/1

== system TrajectoryGenerator3DOF/Trajectory Generator14/M12 ==
  x : Inport
  Discrete FIR Filter1 : DiscreteFir  Coefficients=1/N/Ts*[1 zeros(1,N-1) -1]  InitialStates=Q0  SampleTime=Ts
  Discrete Filter : DiscreteFilter  Numerator=[0 Ts]  Denominator=[1 -1]  InitialStates=Q0  SampleTime=Ts
  y : Outport
  dy : Outport  Port=2
  wires:
  Discrete FIR Filter1/1 -> Discrete Filter/1, dy/1
  x/1 -> Discrete FIR Filter1/1
  Discrete Filter/1 -> y/1

== system TrajectoryGenerator3DOF/Trajectory Generator14/M13 ==
  x : Inport
  Discrete FIR Filter1 : DiscreteFir  Coefficients=1/N/Ts*[1 zeros(1,N-1) -1]  InitialStates=Q0  SampleTime=Ts
  Discrete Filter : DiscreteFilter  Numerator=[0 Ts]  Denominator=[1 -1]  InitialStates=Q0  SampleTime=Ts
  y : Outport
  dy : Outport  Port=2
  wires:
  Discrete FIR Filter1/1 -> Discrete Filter/1, dy/1
  x/1 -> Discrete FIR Filter1/1
  Discrete Filter/1 -> y/1

== system TrajectoryGenerator3DOF/Trajectory Generator14/M14 ==
  x : Inport
  Discrete FIR Filter1 : DiscreteFir  Coefficients=1/N/Ts*[1 zeros(1,N-1) -1]  InitialStates=Q0  SampleTime=Ts
  Discrete Filter : DiscreteFilter  Numerator=[0 Ts]  Denominator=[1 -1]  InitialStates=Q0  SampleTime=Ts
  y : Outport
  dy : Outport  Port=2
  wires:
  Discrete FIR Filter1/1 -> Discrete Filter/1, dy/1
  x/1 -> Discrete FIR Filter1/1
  Discrete Filter/1 -> y/1

== system TrajectoryGenerator3DOF/Trajectory Generator14/M22 ==
  x : Inport
  Discrete FIR Filter1 : DiscreteFir  Coefficients=1/N/Ts*[1 zeros(1,N-1) -1]  InitialStates=Q0  SampleTime=Ts
  Discrete Filter : DiscreteFilter  Numerator=[0 Ts]  Denominator=[1 -1]  InitialStates=Q0  SampleTime=Ts
  y : Outport
  dy : Outport  Port=2
  wires:
  Discrete FIR Filter1/1 -> Discrete Filter/1, dy/1
  x/1 -> Discrete FIR Filter1/1
  Discrete Filter/1 -> y/1

== system TrajectoryGenerator3DOF/Trajectory Generator14/M23 ==
  x : Inport
  Discrete FIR Filter1 : DiscreteFir  Coefficients=1/N/Ts*[1 zeros(1,N-1) -1]  InitialStates=Q0  SampleTime=Ts
  Discrete Filter : DiscreteFilter  Numerator=[0 Ts]  Denominator=[1 -1]  InitialStates=Q0  SampleTime=Ts
  y : Outport
  dy : Outport  Port=2
  wires:
  Discrete FIR Filter1/1 -> Discrete Filter/1, dy/1
  x/1 -> Discrete FIR Filter1/1
  Discrete Filter/1 -> y/1

== system TrajectoryGenerator3DOF/Trajectory Generator14/M24 ==
  x : Inport
  Discrete FIR Filter1 : DiscreteFir  Coefficients=1/N/Ts*[1 zeros(1,N-1) -1]  InitialStates=Q0  SampleTime=Ts
  Discrete Filter : DiscreteFilter  Numerator=[0 Ts]  Denominator=[1 -1]  InitialStates=Q0  SampleTime=Ts
  y : Outport
  dy : Outport  Port=2
  wires:
  Discrete FIR Filter1/1 -> Discrete Filter/1, dy/1
  x/1 -> Discrete FIR Filter1/1
  Discrete Filter/1 -> y/1

== system TrajectoryGenerator3DOF/Trajectory Generator14/M33 ==
  x : Inport
  Discrete FIR Filter1 : DiscreteFir  Coefficients=1/N/Ts*[1 zeros(1,N-1) -1]  InitialStates=Q0  SampleTime=Ts
  Discrete Filter : DiscreteFilter  Numerator=[0 Ts]  Denominator=[1 -1]  InitialStates=Q0  SampleTime=Ts
  y : Outport
  dy : Outport  Port=2
  wires:
  Discrete FIR Filter1/1 -> Discrete Filter/1, dy/1
  x/1 -> Discrete FIR Filter1/1
  Discrete Filter/1 -> y/1

== system TrajectoryGenerator3DOF/Trajectory Generator14/M34 ==
  x : Inport
  Discrete FIR Filter1 : DiscreteFir  Coefficients=1/N/Ts*[1 zeros(1,N-1) -1]  InitialStates=Q0  SampleTime=Ts
  Discrete Filter : DiscreteFilter  Numerator=[0 Ts]  Denominator=[1 -1]  InitialStates=Q0  SampleTime=Ts
  y : Outport
  dy : Outport  Port=2
  wires:
  Discrete FIR Filter1/1 -> Discrete Filter/1, dy/1
  x/1 -> Discrete FIR Filter1/1
  Discrete Filter/1 -> y/1

== system TrajectoryGenerator3DOF/Trajectory Generator14/M44 ==
  x : Inport
  Discrete FIR Filter1 : DiscreteFir  Coefficients=1/N/Ts*[1 zeros(1,N-1) -1]  InitialStates=Q0  SampleTime=Ts
  Discrete Filter : DiscreteFilter  Numerator=[0 Ts]  Denominator=[1 -1]  InitialStates=Q0  SampleTime=Ts
  y : Outport
  dy : Outport  Port=2
  wires:
  Discrete FIR Filter1/1 -> Discrete Filter/1, dy/1
  x/1 -> Discrete FIR Filter1/1
  Discrete Filter/1 -> y/1

== system TrajectoryGenerator3DOF/Trajectory Generator15/M11 ==
  x : Inport
  Discrete FIR Filter1 : DiscreteFir  Coefficients=1/N/Ts*[1 zeros(1,N-1) -1]  InitialStates=Q0  SampleTime=Ts
  Discrete Filter : DiscreteFilter  Numerator=[0 Ts]  Denominator=[1 -1]  InitialStates=Q0  SampleTime=Ts
  y : Outport
  dy : Outport  Port=2
  wires:
  Discrete FIR Filter1/1 -> Discrete Filter/1, dy/1
  x/1 -> Discrete FIR Filter1/1
  Discrete Filter/1 -> y/1

== system TrajectoryGenerator3DOF/Trajectory Generator15/M12 ==
  x : Inport
  Discrete FIR Filter1 : DiscreteFir  Coefficients=1/N/Ts*[1 zeros(1,N-1) -1]  InitialStates=Q0  SampleTime=Ts
  Discrete Filter : DiscreteFilter  Numerator=[0 Ts]  Denominator=[1 -1]  InitialStates=Q0  SampleTime=Ts
  y : Outport
  dy : Outport  Port=2
  wires:
  Discrete FIR Filter1/1 -> Discrete Filter/1, dy/1
  x/1 -> Discrete FIR Filter1/1
  Discrete Filter/1 -> y/1

== system TrajectoryGenerator3DOF/Trajectory Generator15/M13 ==
  x : Inport
  Discrete FIR Filter1 : DiscreteFir  Coefficients=1/N/Ts*[1 zeros(1,N-1) -1]  InitialStates=Q0  SampleTime=Ts
  Discrete Filter : DiscreteFilter  Numerator=[0 Ts]  Denominator=[1 -1]  InitialStates=Q0  SampleTime=Ts
  y : Outport
  dy : Outport  Port=2
  wires:
  Discrete FIR Filter1/1 -> Discrete Filter/1, dy/1
  x/1 -> Discrete FIR Filter1/1
  Discrete Filter/1 -> y/1

== system TrajectoryGenerator3DOF/Trajectory Generator15/M14 ==
  x : Inport
  Discrete FIR Filter1 : DiscreteFir  Coefficients=1/N/Ts*[1 zeros(1,N-1) -1]  InitialStates=Q0  SampleTime=Ts
  Discrete Filter : DiscreteFilter  Numerator=[0 Ts]  Denominator=[1 -1]  InitialStates=Q0  SampleTime=Ts
  y : Outport
  dy : Outport  Port=2
  wires:
  Discrete FIR Filter1/1 -> Discrete Filter/1, dy/1
  x/1 -> Discrete FIR Filter1/1
  Discrete Filter/1 -> y/1

== system TrajectoryGenerator3DOF/Trajectory Generator15/M22 ==
  x : Inport
  Discrete FIR Filter1 : DiscreteFir  Coefficients=1/N/Ts*[1 zeros(1,N-1) -1]  InitialStates=Q0  SampleTime=Ts
  Discrete Filter : DiscreteFilter  Numerator=[0 Ts]  Denominator=[1 -1]  InitialStates=Q0  SampleTime=Ts
  y : Outport
  dy : Outport  Port=2
  wires:
  Discrete FIR Filter1/1 -> Discrete Filter/1, dy/1
  x/1 -> Discrete FIR Filter1/1
  Discrete Filter/1 -> y/1

== system TrajectoryGenerator3DOF/Trajectory Generator15/M23 ==
  x : Inport
  Discrete FIR Filter1 : DiscreteFir  Coefficients=1/N/Ts*[1 zeros(1,N-1) -1]  InitialStates=Q0  SampleTime=Ts
  Discrete Filter : DiscreteFilter  Numerator=[0 Ts]  Denominator=[1 -1]  InitialStates=Q0  SampleTime=Ts
  y : Outport
  dy : Outport  Port=2
  wires:
  Discrete FIR Filter1/1 -> Discrete Filter/1, dy/1
  x/1 -> Discrete FIR Filter1/1
  Discrete Filter/1 -> y/1

== system TrajectoryGenerator3DOF/Trajectory Generator15/M24 ==
  x : Inport
  Discrete FIR Filter1 : DiscreteFir  Coefficients=1/N/Ts*[1 zeros(1,N-1) -1]  InitialStates=Q0  SampleTime=Ts
  Discrete Filter : DiscreteFilter  Numerator=[0 Ts]  Denominator=[1 -1]  InitialStates=Q0  SampleTime=Ts
  y : Outport
  dy : Outport  Port=2
  wires:
  Discrete FIR Filter1/1 -> Discrete Filter/1, dy/1
  x/1 -> Discrete FIR Filter1/1
  Discrete Filter/1 -> y/1

== system TrajectoryGenerator3DOF/Trajectory Generator15/M33 ==
  x : Inport
  Discrete FIR Filter1 : DiscreteFir  Coefficients=1/N/Ts*[1 zeros(1,N-1) -1]  InitialStates=Q0  SampleTime=Ts
  Discrete Filter : DiscreteFilter  Numerator=[0 Ts]  Denominator=[1 -1]  InitialStates=Q0  SampleTime=Ts
  y : Outport
  dy : Outport  Port=2
  wires:
  Discrete FIR Filter1/1 -> Discrete Filter/1, dy/1
  x/1 -> Discrete FIR Filter1/1
  Discrete Filter/1 -> y/1

== system TrajectoryGenerator3DOF/Trajectory Generator15/M34 ==
  x : Inport
  Discrete FIR Filter1 : DiscreteFir  Coefficients=1/N/Ts*[1 zeros(1,N-1) -1]  InitialStates=Q0  SampleTime=Ts
  Discrete Filter : DiscreteFilter  Numerator=[0 Ts]  Denominator=[1 -1]  InitialStates=Q0  SampleTime=Ts
  y : Outport
  dy : Outport  Port=2
  wires:
  Discrete FIR Filter1/1 -> Discrete Filter/1, dy/1
  x/1 -> Discrete FIR Filter1/1
  Discrete Filter/1 -> y/1

== system TrajectoryGenerator3DOF/Trajectory Generator15/M44 ==
  x : Inport
  Discrete FIR Filter1 : DiscreteFir  Coefficients=1/N/Ts*[1 zeros(1,N-1) -1]  InitialStates=Q0  SampleTime=Ts
  Discrete Filter : DiscreteFilter  Numerator=[0 Ts]  Denominator=[1 -1]  InitialStates=Q0  SampleTime=Ts
  y : Outport
  dy : Outport  Port=2
  wires:
  Discrete FIR Filter1/1 -> Discrete Filter/1, dy/1
  x/1 -> Discrete FIR Filter1/1
  Discrete Filter/1 -> y/1

== system TrajectoryGenerator3DOF/Trajectory Generator16/M11 ==
  x : Inport
  Discrete FIR Filter1 : DiscreteFir  Coefficients=1/N/Ts*[1 zeros(1,N-1) -1]  InitialStates=Q0  SampleTime=Ts
  Discrete Filter : DiscreteFilter  Numerator=[0 Ts]  Denominator=[1 -1]  InitialStates=Q0  SampleTime=Ts
  y : Outport
  dy : Outport  Port=2
  wires:
  Discrete FIR Filter1/1 -> Discrete Filter/1, dy/1
  x/1 -> Discrete FIR Filter1/1
  Discrete Filter/1 -> y/1

== system TrajectoryGenerator3DOF/Trajectory Generator16/M12 ==
  x : Inport
  Discrete FIR Filter1 : DiscreteFir  Coefficients=1/N/Ts*[1 zeros(1,N-1) -1]  InitialStates=Q0  SampleTime=Ts
  Discrete Filter : DiscreteFilter  Numerator=[0 Ts]  Denominator=[1 -1]  InitialStates=Q0  SampleTime=Ts
  y : Outport
  dy : Outport  Port=2
  wires:
  Discrete FIR Filter1/1 -> Discrete Filter/1, dy/1
  x/1 -> Discrete FIR Filter1/1
  Discrete Filter/1 -> y/1

== system TrajectoryGenerator3DOF/Trajectory Generator16/M13 ==
  x : Inport
  Discrete FIR Filter1 : DiscreteFir  Coefficients=1/N/Ts*[1 zeros(1,N-1) -1]  InitialStates=Q0  SampleTime=Ts
  Discrete Filter : DiscreteFilter  Numerator=[0 Ts]  Denominator=[1 -1]  InitialStates=Q0  SampleTime=Ts
  y : Outport
  dy : Outport  Port=2
  wires:
  Discrete FIR Filter1/1 -> Discrete Filter/1, dy/1
  x/1 -> Discrete FIR Filter1/1
  Discrete Filter/1 -> y/1

== system TrajectoryGenerator3DOF/Trajectory Generator16/M14 ==
  x : Inport
  Discrete FIR Filter1 : DiscreteFir  Coefficients=1/N/Ts*[1 zeros(1,N-1) -1]  InitialStates=Q0  SampleTime=Ts
  Discrete Filter : DiscreteFilter  Numerator=[0 Ts]  Denominator=[1 -1]  InitialStates=Q0  SampleTime=Ts
  y : Outport
  dy : Outport  Port=2
  wires:
  Discrete FIR Filter1/1 -> Discrete Filter/1, dy/1
  x/1 -> Discrete FIR Filter1/1
  Discrete Filter/1 -> y/1

== system TrajectoryGenerator3DOF/Trajectory Generator16/M22 ==
  x : Inport
  Discrete FIR Filter1 : DiscreteFir  Coefficients=1/N/Ts*[1 zeros(1,N-1) -1]  InitialStates=Q0  SampleTime=Ts
  Discrete Filter : DiscreteFilter  Numerator=[0 Ts]  Denominator=[1 -1]  InitialStates=Q0  SampleTime=Ts
  y : Outport
  dy : Outport  Port=2
  wires:
  Discrete FIR Filter1/1 -> Discrete Filter/1, dy/1
  x/1 -> Discrete FIR Filter1/1
  Discrete Filter/1 -> y/1

== system TrajectoryGenerator3DOF/Trajectory Generator16/M23 ==
  x : Inport
  Discrete FIR Filter1 : DiscreteFir  Coefficients=1/N/Ts*[1 zeros(1,N-1) -1]  InitialStates=Q0  SampleTime=Ts
  Discrete Filter : DiscreteFilter  Numerator=[0 Ts]  Denominator=[1 -1]  InitialStates=Q0  SampleTime=Ts
  y : Outport
  dy : Outport  Port=2
  wires:
  Discrete FIR Filter1/1 -> Discrete Filter/1, dy/1
  x/1 -> Discrete FIR Filter1/1
  Discrete Filter/1 -> y/1

== system TrajectoryGenerator3DOF/Trajectory Generator16/M24 ==
  x : Inport
  Discrete FIR Filter1 : DiscreteFir  Coefficients=1/N/Ts*[1 zeros(1,N-1) -1]  InitialStates=Q0  SampleTime=Ts
  Discrete Filter : DiscreteFilter  Numerator=[0 Ts]  Denominator=[1 -1]  InitialStates=Q0  SampleTime=Ts
  y : Outport
  dy : Outport  Port=2
  wires:
  Discrete FIR Filter1/1 -> Discrete Filter/1, dy/1
  x/1 -> Discrete FIR Filter1/1
  Discrete Filter/1 -> y/1

== system TrajectoryGenerator3DOF/Trajectory Generator16/M33 ==
  x : Inport
  Discrete FIR Filter1 : DiscreteFir  Coefficients=1/N/Ts*[1 zeros(1,N-1) -1]  InitialStates=Q0  SampleTime=Ts
  Discrete Filter : DiscreteFilter  Numerator=[0 Ts]  Denominator=[1 -1]  InitialStates=Q0  SampleTime=Ts
  y : Outport
  dy : Outport  Port=2
  wires:
  Discrete FIR Filter1/1 -> Discrete Filter/1, dy/1
  x/1 -> Discrete FIR Filter1/1
  Discrete Filter/1 -> y/1

== system TrajectoryGenerator3DOF/Trajectory Generator16/M34 ==
  x : Inport
  Discrete FIR Filter1 : DiscreteFir  Coefficients=1/N/Ts*[1 zeros(1,N-1) -1]  InitialStates=Q0  SampleTime=Ts
  Discrete Filter : DiscreteFilter  Numerator=[0 Ts]  Denominator=[1 -1]  InitialStates=Q0  SampleTime=Ts
  y : Outport
  dy : Outport  Port=2
  wires:
  Discrete FIR Filter1/1 -> Discrete Filter/1, dy/1
  x/1 -> Discrete FIR Filter1/1
  Discrete Filter/1 -> y/1

== system TrajectoryGenerator3DOF/Trajectory Generator16/M44 ==
  x : Inport
  Discrete FIR Filter1 : DiscreteFir  Coefficients=1/N/Ts*[1 zeros(1,N-1) -1]  InitialStates=Q0  SampleTime=Ts
  Discrete Filter : DiscreteFilter  Numerator=[0 Ts]  Denominator=[1 -1]  InitialStates=Q0  SampleTime=Ts
  y : Outport
  dy : Outport  Port=2
  wires:
  Discrete FIR Filter1/1 -> Discrete Filter/1, dy/1
  x/1 -> Discrete FIR Filter1/1
  Discrete Filter/1 -> y/1

== system TrajectoryGenerator3DOF/Trajectory Generator17/M11 ==
  x : Inport
  Discrete FIR Filter1 : DiscreteFir  Coefficients=1/N/Ts*[1 zeros(1,N-1) -1]  InitialStates=Q0  SampleTime=Ts
  Discrete Filter : DiscreteFilter  Numerator=[0 Ts]  Denominator=[1 -1]  InitialStates=Q0  SampleTime=Ts
  y : Outport
  dy : Outport  Port=2
  wires:
  Discrete FIR Filter1/1 -> Discrete Filter/1, dy/1
  x/1 -> Discrete FIR Filter1/1
  Discrete Filter/1 -> y/1

== system TrajectoryGenerator3DOF/Trajectory Generator17/M12 ==
  x : Inport
  Discrete FIR Filter1 : DiscreteFir  Coefficients=1/N/Ts*[1 zeros(1,N-1) -1]  InitialStates=Q0  SampleTime=Ts
  Discrete Filter : DiscreteFilter  Numerator=[0 Ts]  Denominator=[1 -1]  InitialStates=Q0  SampleTime=Ts
  y : Outport
  dy : Outport  Port=2
  wires:
  Discrete FIR Filter1/1 -> Discrete Filter/1, dy/1
  x/1 -> Discrete FIR Filter1/1
  Discrete Filter/1 -> y/1

== system TrajectoryGenerator3DOF/Trajectory Generator17/M13 ==
  x : Inport
  Discrete FIR Filter1 : DiscreteFir  Coefficients=1/N/Ts*[1 zeros(1,N-1) -1]  InitialStates=Q0  SampleTime=Ts
  Discrete Filter : DiscreteFilter  Numerator=[0 Ts]  Denominator=[1 -1]  InitialStates=Q0  SampleTime=Ts
  y : Outport
  dy : Outport  Port=2
  wires:
  Discrete FIR Filter1/1 -> Discrete Filter/1, dy/1
  x/1 -> Discrete FIR Filter1/1
  Discrete Filter/1 -> y/1

== system TrajectoryGenerator3DOF/Trajectory Generator17/M14 ==
  x : Inport
  Discrete FIR Filter1 : DiscreteFir  Coefficients=1/N/Ts*[1 zeros(1,N-1) -1]  InitialStates=Q0  SampleTime=Ts
  Discrete Filter : DiscreteFilter  Numerator=[0 Ts]  Denominator=[1 -1]  InitialStates=Q0  SampleTime=Ts
  y : Outport
  dy : Outport  Port=2
  wires:
  Discrete FIR Filter1/1 -> Discrete Filter/1, dy/1
  x/1 -> Discrete FIR Filter1/1
  Discrete Filter/1 -> y/1
